simulink model "hw7plots"  (R2022b)
settings: Solver=VariableStepAuto  StartTime=0.0  StopTime=1800  RelTol=1e-3
libraries: simulink_extras x1
settings Model: Creator=izacu  LastModifiedBy=izacu

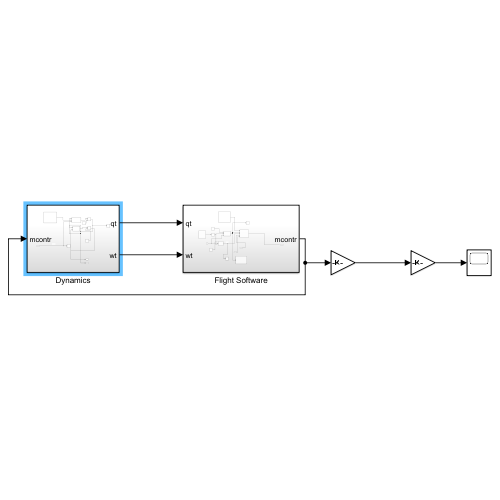
[thumbnail: Simulink's stored preview of the top-level diagram]
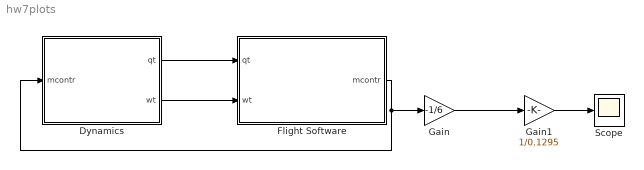
== system hw7plots ==
  Dynamics : Subsystem
  Flight Software : Subsystem
  Gain : Gain  Gain=-1/6
  Gain1 : Gain  Gain=1/0.1295
  Scope : Scope
  wires:
  Dynamics/1(qt) -> Flight Software/1(qt)
  Dynamics/2(wt) -> Flight Software/2(wt)
  Flight Software/1(mcontr) -> Gain/1, Dynamics/1(mcontr)
  Gain/1 -> Gain1/1
  Gain1/1 -> Scope/1

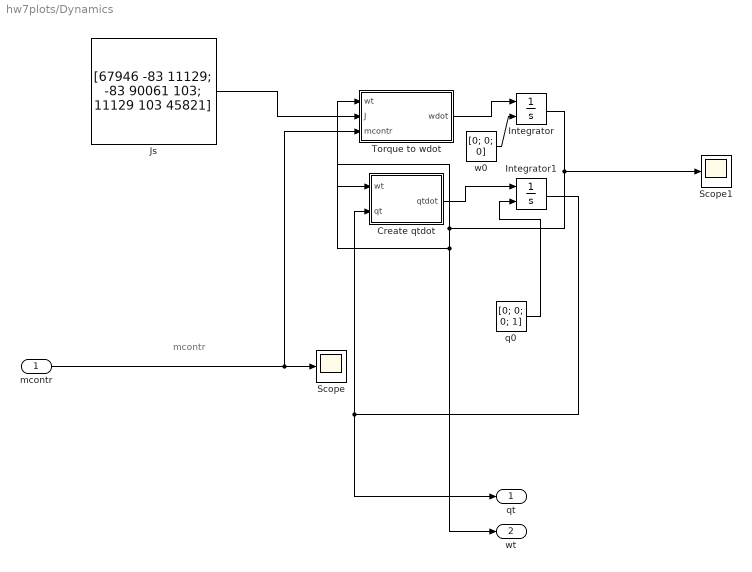
== system hw7plots/Dynamics ==
  note: mcontr
  mcontr : Inport
  Create qtdot : MATLAB Function  TreatAsAtomicUnit=on
  Integrator : Integrator  InitialConditionSource=external
  Integrator1 : Integrator  InitialConditionSource=external
  Js : Constant  Value=[67946 -83 11129; -83 90061 103; 11129 103 45821]
  Scope : Scope
  Scope1 : Scope
  Torque to wdot : MATLAB Function  TreatAsAtomicUnit=on
  q0 : Constant  Value=[0; 0; 0; 1]
  w0 : Constant  Value=[0; 0; 0]
  qt : Outport
  wt : Outport  Port=2
  wires:
  Integrator1/1 -> qt/1, Create qtdot/2(qt)
  Integrator/1 -> Scope1/1, wt/1, Torque to wdot/1(wt), Create qtdot/1(wt)
  Create qtdot/1(qtdot) -> Integrator1/1
  Torque to wdot/1(wdot) -> Integrator/1
  q0/1 -> Integrator1/2
  Js/1 -> Torque to wdot/2(J)
  w0/1 -> Integrator/2
  mcontr/1 -> Scope/1, Torque to wdot/3(mcontr)

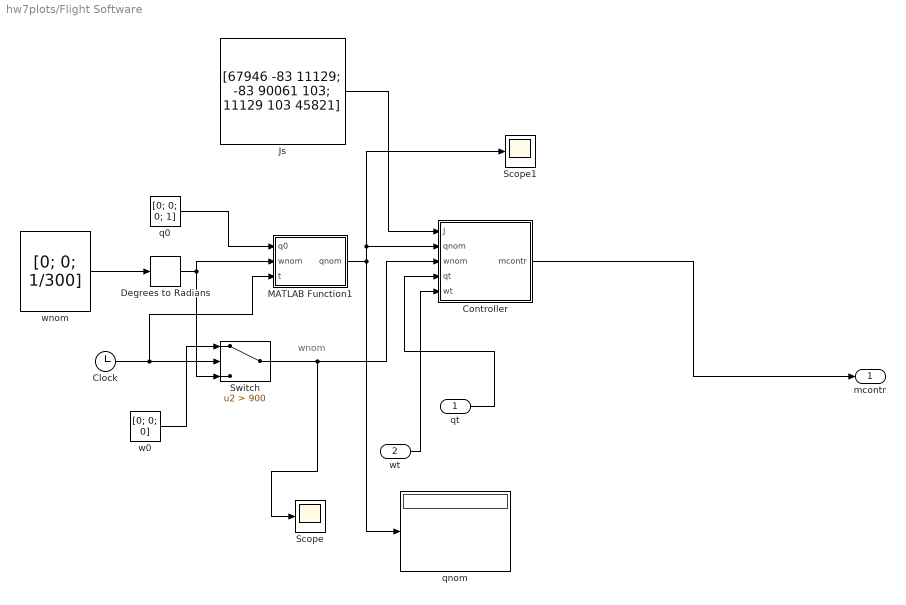
== system hw7plots/Flight Software ==
  note: wnom
  qt : Inport
  wt : Inport  Port=2
  Clock : Clock
  Controller : MATLAB Function  TreatAsAtomicUnit=on
  Degrees to Radians : simulink_extras/Transformations/Degrees to Radians
  Js : Constant  Value=[67946 -83 11129; -83 90061 103; 11129 103 45821]
  MATLAB Function1 : MATLAB Function  TreatAsAtomicUnit=on
  Scope : Scope
  Scope1 : Scope
  Switch : Switch  Criteria=u2 > Threshold  Threshold=900  SaturateOnIntegerOverflow=off  InputSameDT=off
  q0 : Constant  Value=[0; 0; 0; 1]
  qnom : Display
  w0 : Constant  Value=[0; 0; 0]
  wnom : Constant  Value=[0; 0; 1/300]
  mcontr : Outport
  wires:
  wnom/1 -> Degrees to Radians/1
  q0/1 -> MATLAB Function1/1(q0)
  Degrees to Radians/1 -> Switch/3, MATLAB Function1/2(wnom)
  Js/1 -> Controller/1(J)
  MATLAB Function1/1(qnom) -> Scope1/1, Controller/2(qnom), qnom/1
  Clock/1 -> MATLAB Function1/3(t), Switch/2
  Switch/1 -> Scope/1, Controller/3(wnom)
  wt/1 -> Controller/5(wt)
  qt/1 -> Controller/4(qt)
  w0/1 -> Switch/1
  Controller/1(mcontr) -> mcontr/1

== matlab function hw7plots/Flight Software/MATLAB Function1 ==
  data: q0 input; qnom output; wnom input; t input
function qnom = fcn(q0,wnom,t)
if t < 900
    thetatot = norm(wnom)*t;
else
    thetatot = norm(wnom)*900;
end
e = wnom ./ norm(wnom);

qtotv = sin(thetatot/2)*e;
qtots = cos(thetatot/2);

qtot = [qtotv; qtots];

qnom = qmult(qtot,q0);



function q3 = qmult(q2,q1)

q3 = [q2(4).*q1(1:3) + q1(4).*q2(1:3) - cross(q2(1:3),q1(1:3));
    q2(4)*q1(4) - dot(q2(1:3),q1(1:3))];

== matlab function hw7plots/Flight Software/Controller ==
  data: J input; qnom input; mcontr output; wnom input; qt input; wt input
function mcontr = fcn(J,qnom,wnom,qt,wt)

qtconj = qt;
qtconj(1:3) = -qt(1:3);
qerr = qmult(qnom,qtconj);

error = (2/qerr(4))*qerr(1:3);

werr = wnom - wt;

derror = -skewsymmetric(wnom)*error + werr;

Kd = 0.1;
Kp = 0.1;

u = Kd*derror + Kp*error;

mcontr = J*u;

end
function q3 = qmult(q2,q1)

q3 = [q2(4).*q1(1:3) + q1(4).*q2(1:3) - cross(q2(1:3),q1(1:3));
    q2(4)*q1(4) - dot(q2(1:3),q1(1:3))];

end

function ssmatrix = skewsymmetric(vector)

ssmatrix = [0 -vector(3) vector(2);
            vector(3) 0 -vector(1);
            -vector(2) vector(1) 0];

end

== matlab function hw7plots/Dynamics/Torque to wdot ==
  data: wt input; wdot output; J input; mcontr input
function wdot = fcn(wt,J,mcontr)

wdot = inv(J)*(mcontr - cross(wt, J*wt));

== matlab function hw7plots/Dynamics/Create qtdot ==
  data: wt input; qtdot output; qt input
function qtdot = fcn(wt,qt)
v1 = zeros(4,1);
v1(1:3) = wt;
v1(4) = 0;
qtdot = qmult(0.5 * v1, qt);



end



function q3 = qmult(q2,q1)

q3 = [q2(4).*q1(1:3) + q1(4).*q2(1:3) - cross(q2(1:3),q1(1:3));
    q2(4)*q1(4) - dot(q2(1:3),q1(1:3))];

end
